simulink library "unpartitionedFluidLoads"  (R2020a)
settings: Solver=VariableStepAuto  StartTime=0.0  StopTime=10.0  RelTol=1e-3
values from neighbouring files (symbols this model uses):
  fluidDensity = 1000    [fluidDynamicSurface_ts.m]
undefined symbols (not defined in the file or in its folder): fluidMomentArms, fluidRefArea, vcl, wingTips
libraries: vrlib x3, dynamicPressure_ul x1, eeGeneralControl x1, Copy_of_clAndCdCalculator_cl x1, alphaBetaLE_ul x1, localApparentWind_ul x1, rotateAboutVec x1
settings Model: Creator=Ayaz  LastModifiedBy=adabney

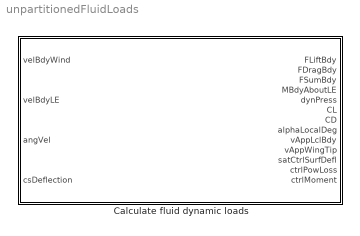
== system unpartitionedFluidLoads ==
  Calculate fluid dynamic loads : Subsystem  mask{aSurf=vcl.portWing, sRef=fluidRefArea, rArm_LE=fluidMomentArms(:,1), rTip_LE=wingTips(:,1), fluidDensity=fluidDensity}
      mask prompts: aSurf "Aerosurf object"; sRef "Reference area"; rArm_LE "Moment arm wrt wing LE"; rTip_LE "Surface tip wrt wing LE"; fluidDensity "Fluid density"

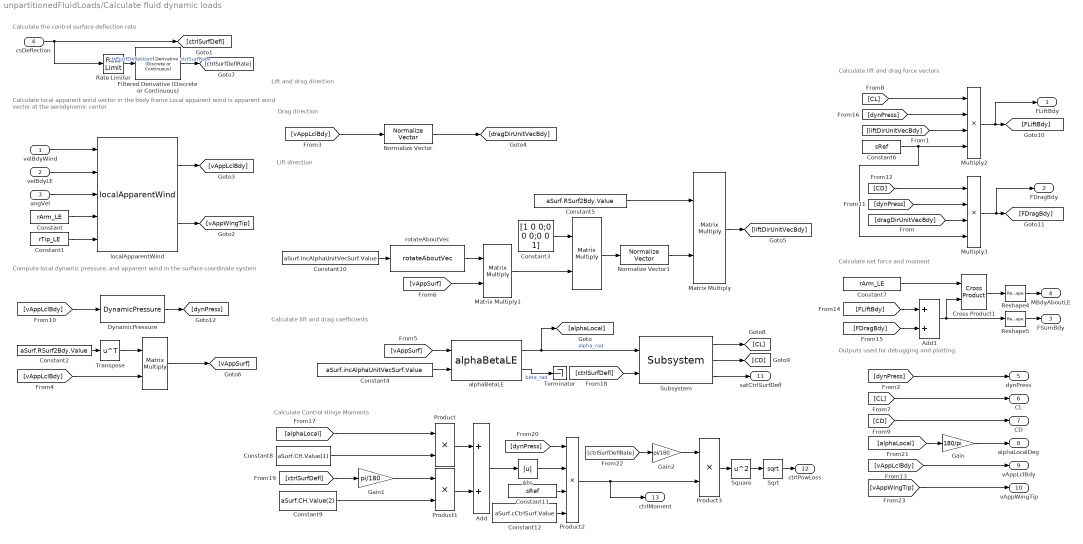
== system unpartitionedFluidLoads/Calculate fluid dynamic loads ==
  note: Calculate Control Hinge Moments
  note: Calculate the control surface deflection rate
  note: Lift and drag direction
  note: Lift direction
  note: Drag direction
  note: Compute local dynamic pressure,
      | and apparent wind in the surface coordinate system
  note: Calculate local apparent wind vector in the body frame
      | Local apparent wind is apparent wind vector at the aerodynamic center
  note: Calculate lift and drag coefficients
  note: Calculate net force and moment
  note: Outputs used for debugging and plotting.
  note: Calculate lift and drag force vectors
  velBdyWind : Inport
  velBdyLE : Inport  Port=2
  angVel : Inport  Port=3
  csDeflection : Inport  Port=4
  " " : Product  Multiplication=Matrix(*)
  "  " : Product  Multiplication=Matrix(*)
  Abs : Abs
  Add : Sum
  Add1 : Sum
  Constant : Constant  Value=rArm_LE  VectorParams1D=off
  Constant1 : Constant  Value=rTip_LE  VectorParams1D=off
  Constant10 : Constant  Value=aSurf.incAlphaUnitVecSurf.Value  VectorParams1D=off
  Constant11 : Constant  Value=sRef
  Constant12 : Constant  Value=aSurf.cCtrlSurf.Value
  Constant2 : Constant  Value=aSurf.RSurf2Bdy.Value  VectorParams1D=off
  Constant3 : Constant  Value=[1 0 0;0 0 0;0 0 1]  VectorParams1D=off
  Constant4 : Constant  Value=aSurf.incAlphaUnitVecSurf.Value  VectorParams1D=off
  Constant5 : Constant  Value=aSurf.RSurf2Bdy.Value  VectorParams1D=off
  Constant6 : Constant  Value=sRef
  Constant7 : Constant  Value=rArm_LE  VectorParams1D=off
  Constant8 : Constant  Value=aSurf.CH.Value(1)
  Constant9 : Constant  Value=aSurf.CH.Value(2)
  Cross Product1 : vrlib/Utilities/Cross Product
  DynamicPressure : dynamicPressure_ul/DynamicPressure  rho=fluidDensity
  Filtered Derivative (Discrete or Continuous) : eeGeneralControl/Filtered Derivative (Discrete or Continuous)  K=1  T=.001  B=inf  A=-inf  minRatio=10  init_option=Inherited from block input  x0=0  Ts=-1
      settings: SourceProductBaseCode=PS
  Gain : Gain  Gain=180/pi
  Gain1 : Gain  Gain=pi/180
  Gain2 : Gain  Gain=pi/180
  Matrix Multiply : Product  Multiplication=Matrix(*)
  Matrix Multiply1 : Product  Multiplication=Matrix(*)
  Multiply2 : Product  Inputs=4
  Multiply3 : Product  Inputs=4
  Normalize Vector : vrlib/Utilities/Normalize Vector  maxzero=0
  Normalize Vector1 : vrlib/Utilities/Normalize Vector  maxzero=0
  Product : Product
  Product1 : Product
  Product2 : Product  Inputs=4
  Product3 : Product
  Rate Limiter : RateLimiter  RisingSlewLimit=aSurf.maxCtrlDefSpeed.Value  FallingSlewLimit=-aSurf.maxCtrlDefSpeed.Value  SampleTimeMode=inherited
  Reshape4 : Reshape  OutputDimensionality=Column vector (2-D)
  Reshape5 : Reshape  OutputDimensionality=Column vector (2-D)
  Sqrt : Sqrt  SaturateOnIntegerOverflow=on
  Square : Math  Operator=square  SaturateOnIntegerOverflow=on
  Subsystem : Copy_of_clAndCdCalculator_cl/Subsystem  aSurf=aSurf
  Terminator : Terminator
  Transpose : Math  Operator=transpose  SignedPower=on  SaturateOnIntegerOverflow=on
  alphaBetaLE : alphaBetaLE_ul/alphaBetaLE  SystemSampleTime=-1  Latency=0  AutoFrameSizeCalculation=off
  localApparentWind : localApparentWind_ul/localApparentWind  SystemSampleTime=-1  Latency=0  AutoFrameSizeCalculation=off
  rotateAboutVec : rotateAboutVec/rotateAboutVec  ang=90
  FLiftBdy : Outport  VectorParamsAs1DForOutWhenUnconnected=off
  FDragBdy : Outport  Port=2  VectorParamsAs1DForOutWhenUnconnected=off
  FSumBdy : Outport  Port=3  VectorParamsAs1DForOutWhenUnconnected=off
  MBdyAboutLE : Outport  Port=4  PortDimensions=[3 1]  VectorParamsAs1DForOutWhenUnconnected=off
  dynPress : Outport  Port=5  VectorParamsAs1DForOutWhenUnconnected=off
  CL : Outport  Port=6  VectorParamsAs1DForOutWhenUnconnected=off
  CD : Outport  Port=7  VectorParamsAs1DForOutWhenUnconnected=off
  alphaLocalDeg : Outport  Port=8  VectorParamsAs1DForOutWhenUnconnected=off
  vAppLclBdy : Outport  Port=9  VectorParamsAs1DForOutWhenUnconnected=off
  vAppWingTip : Outport  Port=10  VectorParamsAs1DForOutWhenUnconnected=off
  satCtrlSurfDefl : Outport  Port=11
  ctrlPowLoss : Outport  Port=12
  ctrlMoment : Outport  Port=13
  wires:
  velBdyWind/1 -> localApparentWind/1
  velBdyLE/1 -> localApparentWind/2
  angVel/1 -> localApparentWind/3
  Constant/1 -> localApparentWind/4
  Constant1/1 -> localApparentWind/5
  localApparentWind/1 -> [vAppLclBdy]
  localApparentWind/2 -> [vAppWingTip]
  [vAppLclBdy] -> DynamicPressure/1
  "  "/1 -> [vAppSurf]
  Constant2/1 -> Transpose/1
  [vAppLclBdy] -> "  "/2
  DynamicPressure/1 -> [dynPress]
  Transpose/1 -> "  "/1
  Constant3/1 -> " "/1
  rotateAboutVec/1 -> Matrix Multiply1/1
  Matrix Multiply/1 -> [liftDirUnitVecBdy]
  Normalize Vector1/1 -> Matrix Multiply/2
  Constant10/1 -> rotateAboutVec/1
  Matrix Multiply1/1 -> " "/2
  " "/1 -> Normalize Vector1/1
  Constant5/1 -> Matrix Multiply/1
  [vAppSurf] -> Matrix Multiply1/2
  Normalize Vector/1 -> [dragDirUnitVecBdy]
  [vAppLclBdy] -> Normalize Vector/1
  alphaBetaLE/1 -> [alphaLocal], Subsystem/1  "alpha_rad"
  Constant4/1 -> alphaBetaLE/2
  Subsystem/2 -> [CD]
  alphaBetaLE/2 -> Terminator/1  "beta_rad"
  [ctrlSurfDefl] -> Subsystem/2
  [vAppSurf] -> alphaBetaLE/1
  Subsystem/1 -> [CL]
  Constant6/1 -> Multiply2/4, Multiply3/4
  [vAppLclBdy] -> vAppLclBdy/1
  [dynPress] -> dynPress/1
  [FLiftBdy] -> Add1/1
  [vAppWingTip] -> vAppWingTip/1
  Multiply3/1 -> [FDragBdy], FDragBdy/1
  [dragDirUnitVecBdy] -> Multiply3/3
  [CD] -> CD/1
  [dynPress] -> Multiply2/2
  [alphaLocal] -> Gain/1
  [dynPress] -> Multiply3/2
  [CL] -> CL/1
  [CL] -> Multiply2/1
  [liftDirUnitVecBdy] -> Multiply2/3
  Multiply2/1 -> [FLiftBdy], FLiftBdy/1
  [CD] -> Multiply3/1
  [FDragBdy] -> Add1/2
  Reshape5/1 -> FSumBdy/1
  Cross Product1/1 -> Reshape4/1
  Add1/1 -> Cross Product1/2, Reshape5/1
  Constant7/1 -> Cross Product1/1
  Gain/1 -> alphaLocalDeg/1
  Reshape4/1 -> MBdyAboutLE/1
  Subsystem/3 -> satCtrlSurfDefl/1
  Filtered Derivative (Discrete or Continuous)/1 -> [ctrlSurfDeflRate]  "ctrlSurfRate"
  [alphaLocal] -> Product/1
  Constant8/1 -> Product/2
  [ctrlSurfDefl] -> Gain1/1
  Constant9/1 -> Product1/2
  Product1/1 -> Add/2
  Product/1 -> Add/1
  Add/1 -> Abs/1
  [dynPress] -> Product2/1
  Constant11/1 -> Product2/3
  Constant12/1 -> Product2/4
  Product2/1 -> ctrlMoment/1, Product3/2
  [ctrlSurfDeflRate] -> Gain2/1
  Abs/1 -> Product2/2
  Gain1/1 -> Product1/1
  Gain2/1 -> Product3/1
  csDeflection/1 -> Rate Limiter/1, [ctrlSurfDefl]
  Rate Limiter/1 -> Filtered Derivative (Discrete or Continuous)/1  "ctrlSurfDeflection"
  Product3/1 -> Square/1
  Square/1 -> Sqrt/1
  Sqrt/1 -> ctrlPowLoss/1
